simulink library "AP_Math"  (R2018b)
settings: Solver=VariableStepAuto  StartTime=0.0  StopTime=10.0  RelTol=1e-3
libraries: $bdroot x1
settings Model: Creator=JCZou  LastModifiedBy=zouji
settings CodeAppCC: StateflowObjectComments=on

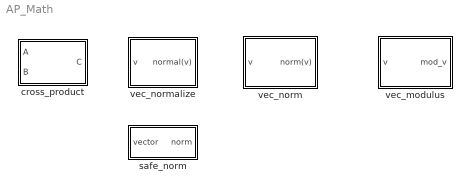
== system AP_Math ==
  cross_product : Subsystem
  safe_norm : Subsystem
  vec_modulus : Subsystem
  vec_norm : Subsystem
  vec_normalize : Subsystem

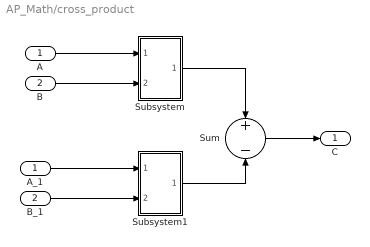
== system AP_Math/cross_product ==
  A : Inport
  B : Inport  Port=2
  A_1 : InportShadow
  B_1 : InportShadow  Port=2
  Subsystem : Subsystem
  Subsystem1 : Subsystem
  Sum : Sum  Inputs=+|-  SaturateOnIntegerOverflow=on  InputSameDT=on  OutDataTypeStr=Inherit: Same as first input
  C : Outport
  wires:
  B/1 -> Subsystem/2(right)
  B_1/1 -> Subsystem1/2(right)
  A/1 -> Subsystem/1(left)
  Subsystem1/1(Out) -> Sum/2
  Sum/1 -> C/1
  Subsystem/1(Out) -> Sum/1
  A_1/1 -> Subsystem1/1(left)

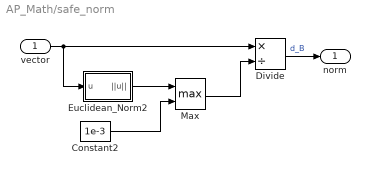
== system AP_Math/safe_norm ==
  vector : Inport
  Constant2 : Constant  Value=1e-3  OutDataTypeStr=Inherit: Inherit via back propagation
  Divide : Product  Inputs=*/
  Euclidean_Norm2 : Subsystem
      mask help: Euclidean Norm
      mask Help: Euclidean Norm
      mask Display: disp('||.||')
  Max : MinMax  Function=max  Inputs=2
  norm : Outport
  wires:
  Max/1 -> Divide/2
  vector/1 -> Divide/1, Euclidean_Norm2/1(u)
  Divide/1 -> norm/1  "d_B"
  Euclidean_Norm2/1(||u||) -> Max/1
  Constant2/1 -> Max/2

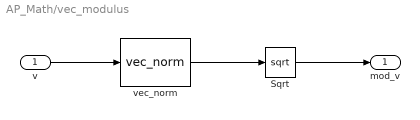
== system AP_Math/vec_modulus ==
  v : Inport
  Sqrt : Sqrt  SaturateOnIntegerOverflow=on
  vec_norm : $bdroot/vec_norm  SystemSampleTime=-1
  mod_v : Outport
  wires:
  v/1 -> vec_norm/1
  vec_norm/1 -> Sqrt/1
  Sqrt/1 -> mod_v/1

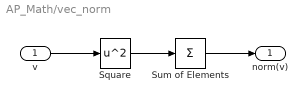
== system AP_Math/vec_norm ==
  v : Inport
  Square : Math  Operator=square  SaturateOnIntegerOverflow=on
  Sum of Elements : Sum  Inputs=+  OutDataTypeStr=Inherit: Same as first input
  norm(v) : Outport
  wires:
  v/1 -> Square/1
  Square/1 -> Sum of Elements/1
  Sum of Elements/1 -> norm(v)/1

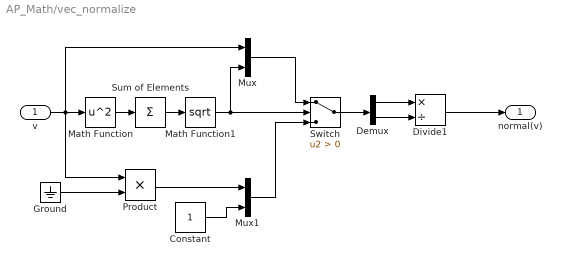
== system AP_Math/vec_normalize ==
  v : Inport
  Constant : Constant  OutDataTypeStr=single
  Demux : Demux  Outputs=[-1 1]
  Divide1 : Product  Inputs=*/  OutDataTypeStr=single
  Ground : Ground
  Math Function : Math  Operator=square  SaturateOnIntegerOverflow=on
  Math Function1 : Math  Operator=sqrt  SaturateOnIntegerOverflow=on
  Mux : Mux  Inputs=2
  Mux1 : Mux  Inputs=2
  Product : Product  OutDataTypeStr=single  RndMeth=Zero
  Sum of Elements : Sum  Inputs=+  AccumDataTypeStr=single
  Switch : Switch  Criteria=u2 > Threshold
  normal(v) : Outport
  wires:
  Sum of Elements/1 -> Math Function1/1
  Mux/1 -> Switch/1
  Switch/1 -> Demux/1
  Ground/1 -> Product/2
  Demux/1 -> Divide1/1
  Math Function1/1 -> Mux/2, Switch/2
  v/1 -> Product/1, Math Function/1, Mux/1
  Math Function/1 -> Sum of Elements/1
  Demux/2 -> Divide1/2
  Product/1 -> Mux1/1
  Mux1/1 -> Switch/3
  Divide1/1 -> normal(v)/1
  Constant/1 -> Mux1/2

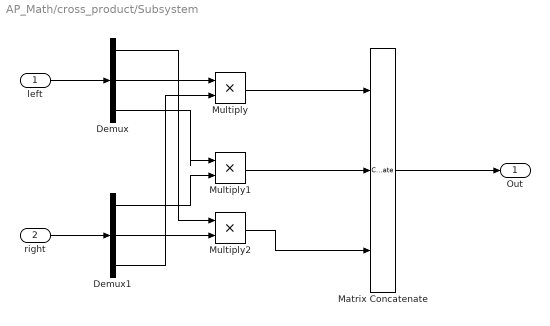
== system AP_Math/cross_product/Subsystem ==
  left : Inport
  right : Inport  Port=2
  Demux : Demux  Outputs=3
  Demux1 : Demux  Outputs=3
  Matrix Concatenate : Concatenate  NumInputs=3  ConcatenateDimension=2
  Multiply : Product  OutDataTypeStr=Inherit: Same as first input
  Multiply1 : Product  OutDataTypeStr=Inherit: Same as first input
  Multiply2 : Product  OutDataTypeStr=Inherit: Same as first input
  Out : Outport
  wires:
  Demux1/1 -> Multiply1/2
  Multiply/1 -> Matrix Concatenate/1
  Demux/3 -> Multiply1/1
  left/1 -> Demux/1
  Multiply1/1 -> Matrix Concatenate/2
  right/1 -> Demux1/1
  Demux1/3 -> Multiply/2
  Matrix Concatenate/1 -> Out/1
  Multiply2/1 -> Matrix Concatenate/3
  Demux/1 -> Multiply2/1
  Demux1/2 -> Multiply2/2
  Demux/2 -> Multiply/1

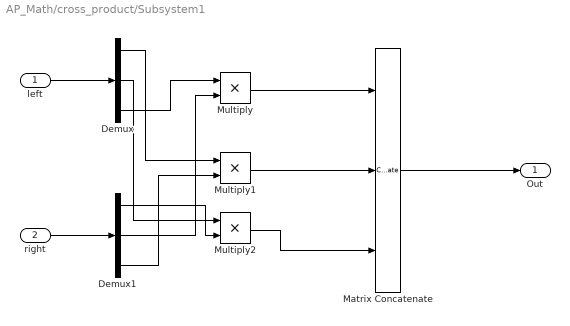
== system AP_Math/cross_product/Subsystem1 ==
  left : Inport
  right : Inport  Port=2
  Demux : Demux  Outputs=3
  Demux1 : Demux  Outputs=3
  Matrix Concatenate : Concatenate  NumInputs=3  ConcatenateDimension=2
  Multiply : Product  OutDataTypeStr=Inherit: Same as first input
  Multiply1 : Product  OutDataTypeStr=Inherit: Same as first input
  Multiply2 : Product  OutDataTypeStr=Inherit: Same as first input
  Out : Outport
  wires:
  Demux/1 -> Multiply1/1
  right/1 -> Demux1/1
  Multiply/1 -> Matrix Concatenate/1
  left/1 -> Demux/1
  Demux1/1 -> Multiply2/2
  Demux/3 -> Multiply/1
  Demux1/2 -> Multiply/2
  Demux1/3 -> Multiply1/2
  Demux/2 -> Multiply2/1
  Multiply1/1 -> Matrix Concatenate/2
  Matrix Concatenate/1 -> Out/1
  Multiply2/1 -> Matrix Concatenate/3

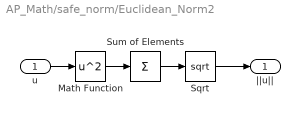
== system AP_Math/safe_norm/Euclidean_Norm2 ==
  u : Inport
  Math Function : Math  Operator=square  SaturateOnIntegerOverflow=on
  Sqrt : Sqrt  SaturateOnIntegerOverflow=on
  Sum of Elements : Sum  Inputs=+
  ||u|| : Outport
  wires:
  Sqrt/1 -> ||u||/1
  Sum of Elements/1 -> Sqrt/1
  Math Function/1 -> Sum of Elements/1
  u/1 -> Math Function/1
